simulink model "Problem_7"  (R2020a)
settings: Solver=VariableStepAuto  StartTime=0.0  StopTime=10.0  RelTol=1e-3
settings Model: Creator=Admin  LastModifiedBy=Admin

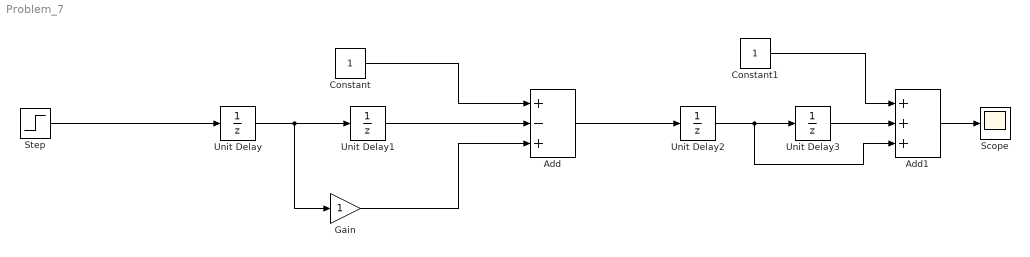
== system Problem_7 ==
  Add : Sum  Inputs=+-+
  Add1 : Sum  Inputs=+++
  Constant : Constant
  Constant1 : Constant
  Gain : Gain
  Scope : Scope
  Step : Step  SampleTime=0
  Unit Delay{,1..3} (4 alike) : UnitDelay  SampleTime=-1  HasFrameUpgradeWarning=on
  wires:
  Unit Delay/1 -> Unit Delay1/1, Gain/1
  Unit Delay2/1 -> Unit Delay3/1, Add1/3
  Step/1 -> Unit Delay/1
  Unit Delay1/1 -> Add/2
  Constant/1 -> Add/1
  Gain/1 -> Add/3
  Constant1/1 -> Add1/1
  Unit Delay3/1 -> Add1/2
  Add1/1 -> Scope/1
  Add/1 -> Unit Delay2/1
